simulink model "untitled"  (R2019a)
settings: Solver=VariableStepAuto  StartTime=0.0  StopTime=1  RelTol=1e-3
values from neighbouring files (symbols this model uses):
  Ts_Control = 5.0000e-05    (= 5e-05)    [Sec_Impedance.m]
  Ts_Power = 5.0000e-05    (= 5e-05)    [Sec_Impedance.m]
undefined symbols (not defined in the file or in its folder): D1, Delta, Ion, Lithium
libraries: powerlib x152, powerlib_meascontrol x65, simulink x14, electricdrivelib x12, simulink_extras x12
(part 2 of 5)

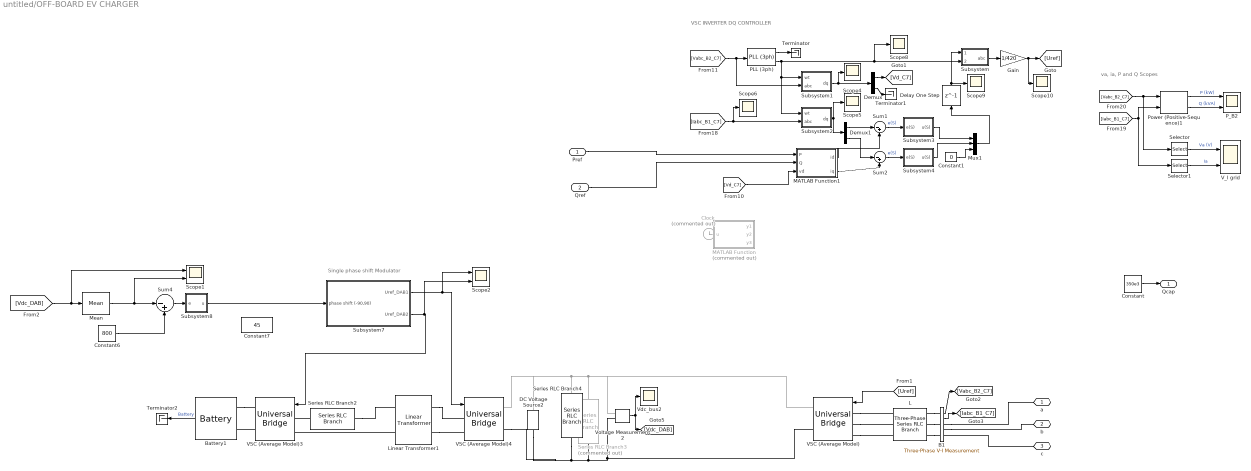
== system untitled/OFF-BOARD EV CHARGER ==
  note: VSC INVERTER DQ CONTROLLER
  note: va, ia, P and Q Scopes
  note: Single phase shift Modulator
  Pref : Inport
  Qref : Inport  Port=2
  B1 : powerlib/Measurements/Three-Phase V-I Measurement  VoltageMeasurement=phase-to-ground  SetLabelV=off  LabelV=Vabc_B1  Vpu=off  VpuLL=off  CurrentMeasurement=yes  SetLabelI=off  LabelI=Iabc_B1_C7  Ipu=off  Pbase=100e6  Vbase=500e3  OutputType=Magnitude  PhasorSimulation=off  PSBequivalent=0
      settings: SourceProductName=Simscape Electrical
  Battery1 : electricdrivelib/Extra Sources/Battery  BatType=Lithium-Ion  ShowTempParam=off  ThermalPreset=no  ShowAgeParam=off  NomV=380  NomQ=5.4*70  SOC=70  Batt_Tr=20  PresetModel=on  MaxQ=378  MinV=285  FullV=442.3151  Dis_rate=164.3478  R=0.010053  Normal_OP=341.8435  expZone="[410.5466       18.5713]"  current=[6.5 13 32.5]  Units=Time  Tci=20  NomT=20  T2=-30  MaxQ2=4.8  FullV2=7.1  Normal_OP2=5.655  expZone2="[6.58           1]"  Rca=0.6  ti=2000  Dp=0  Neq0=0  Tsim=1e6  Ta1=25  Qeol=5.4*0.9  Reol=0.013333*1.2  Char_age=[2.3478, 3]  Dis_age=[2.3478, 10]  N1=1500  N2=10500  N3=1000  N4=1400  Ta2=45  N5=950
      settings: SourceProductName=Simscape Electrical
  Clock : Clock  Commented=on
  Constant : Constant  Value=350e3
  Constant1 : Constant  Value=0
  Constant6 : Constant  Value=800
  Constant7 : Constant  Value=45
  DC Voltage Source2 : powerlib/Electrical Sources/DC Voltage Source  Amplitude=Vdc  Measurements=None
      settings: SourceProductName=Simscape Electrical
  Delay One Step : Delay  DelayLength=1
  Demux : Demux  Outputs=2
  Demux1 : Demux  Outputs=2
  Gain : Gain  Gain=1/420
  L : powerlib/Elements/Three-Phase Series RLC Branch  LConnTagsString=A|B|C  RConnTagsString=A|B|C  BranchType=RL  Resistance=500e-6*377/50/2  Inductance=1200e-6/2  Capacitance=inf  Measurements=None
      settings: SourceProductName=Simscape Electrical
  Linear Transformer1 : powerlib/Elements/Linear Transformer  UNITS=SI  NominalPower=[ 250e3 10000 ]  winding1=[400 0.0032 0.4883e-06]  winding2=[800 0.0032 0.4883e-06]  ThreeWindings=off  winding3=[3.15e+05 19845 2105.6]  RmLm=[800 2.1221]  Measurements=None  DataType=on
      settings: SourceProductName=Simscape Electrical
  MATLAB Function : MATLAB Function  Commented=on  TreatAsAtomicUnit=on
  MATLAB Function1 : MATLAB Function  TreatAsAtomicUnit=on
  Mean : powerlib_meascontrol/Measurements/Mean  Freq=300  Vinit=800  Ts=0
      settings: SourceProductName=Simscape Electrical
  Mux1 : Mux  Inputs=3
  PLL (3ph) : powerlib_meascontrol/PLL/PLL (3ph)  Fmin=58  Par_Init="[-0.57  60]"  ParK=[180, 3200, 1]  TcD=1e-4  MaxRateChangeFreq=12  FilterCutOffFreq=25  Ts=Ts  AGC=on
      settings: SourceProductName=Simscape Electrical
  P_B2 : Scope  NumInputPorts=2
  Power (Positive-Sequence)1 : powerlib_meascontrol/Measurements/Power (Positive-Sequence)  Freq=60  Vinit=[0, 0]  Iinit=[0, 0]  Ts=Ts
      settings: SourceProductName=Simscape Electrical  SourceProductBaseCode=PS
  Scope1 : Scope  NumInputPorts=2
  Scope{4..6,8..10} (6 alike) : Scope
  Scope2 : Scope  NumInputPorts=2
  Selector : Selector  InputPortWidth=3  IndexOptions=Index vector (dialog)  Indices=[1]  OutputSizes=1
  Selector1 : Selector  InputPortWidth=3  IndexOptions=Index vector (dialog)  Indices=[1]  OutputSizes=1
  Series RLC Branch2 : powerlib/Elements/Series RLC Branch  LConnTagsString=__new0  RConnTagsString=__new0  BranchType=L  Resistance=1  Inductance=15e-6  SetiL0=off  InitialCurrent=0  Capacitance=1e-6  Setx0=off  InitialVoltage=0  Measurements=None
      settings: SourceProductName=Simscape Electrical
  Series RLC Branch3 : powerlib/Elements/Series RLC Branch  Commented=on  LConnTagsString=__new0  RConnTagsString=__new0  BranchType=R  Resistance=10  Inductance=1e-3  SetiL0=off  InitialCurrent=0  Capacitance=C  Setx0=off  InitialVoltage=400  Measurements=None
      settings: SourceProductName=Simscape Electrical
  Series RLC Branch4 : powerlib/Elements/Series RLC Branch  LConnTagsString=__new0  RConnTagsString=__new0  BranchType=RC  Resistance=0.1  Inductance=1e-3  SetiL0=off  InitialCurrent=0  Capacitance=C  Setx0=off  InitialVoltage=400  Measurements=None
      settings: SourceProductName=Simscape Electrical
  Subsystem : Subsystem
  Subsystem1 : Subsystem
  Subsystem2 : Subsystem
  Subsystem3 : Subsystem
  Subsystem4 : Subsystem
  Subsystem7 : Subsystem
  Subsystem8 : Subsystem
  Sum1 : Sum  Inputs=|-+
  Sum2 : Sum  Inputs=|-+
  Sum4 : Sum  Inputs=|-+
  Terminator : Terminator
  Terminator1 : Terminator
  Terminator2 : Terminator
  VSC (Average Model) : powerlib/Power Electronics/Universal Bridge  Arms=3  SnubberResistance=1e5  SnubberCapacitance=inf  Device=Average-model based VSC  Ron=1e-3  Lon=0  ForwardVoltages="[  0  0  ]"  ForwardVoltage=0  GTOparameters=[ 10e-6 , 20e-6 ]  IGBTparameters=[ 1e-6 , 2e-6 ]  Measurements=None  Measurements_2=None  converterType=Rectifier
      settings: SourceProductName=Simscape Electrical
  VSC (Average Model)3 : powerlib/Power Electronics/Universal Bridge  Arms=2  SnubberResistance=1e5  SnubberCapacitance=inf  Device=Average-model based VSC  Ron=1e-3  Lon=0  ForwardVoltages="[  0  0  ]"  ForwardVoltage=0  GTOparameters=[ 10e-6 , 20e-6 ]  IGBTparameters=[ 1e-6 , 2e-6 ]  Measurements=None  Measurements_2=None  converterType=Rectifier
      settings: SourceProductName=Simscape Electrical
  VSC (Average Model)4 : powerlib/Power Electronics/Universal Bridge  Arms=2  SnubberResistance=1e5  SnubberCapacitance=inf  Device=Average-model based VSC  Ron=1e-3  Lon=0  ForwardVoltages="[  0  0  ]"  ForwardVoltage=0  GTOparameters=[ 10e-6 , 20e-6 ]  IGBTparameters=[ 1e-6 , 2e-6 ]  Measurements=None  Measurements_2=None  converterType=Rectifier
      settings: SourceProductName=Simscape Electrical
  V_I grid : Scope  NumInputPorts=2
  Vdc_bus2 : Scope
  Voltage Measurement2 : powerlib/Measurements/Voltage Measurement  PhasorSimulation=off  OutputType=Complex  PSBequivalent=0
      settings: SourceProductName=Simscape Electrical
  a : PMIOPort  Side=Right
  b : PMIOPort  Port=2  Side=Right
  c : PMIOPort  Port=3  Side=Right
  Qcap : Outport
  wires:
  Sum2/1 -> Subsystem4/1(e(S))  "e(S)"
  PLL (3ph)/2 -> Subsystem2/1(wt), Subsystem1/1(wt), Scope8/1, Subsystem/2(wt1)
  Mux1/1 -> Delay One Step/1
  Selector/1 -> V_I grid/1  "Va (V)"
  Delay One Step/1 -> Scope9/1, Subsystem/1(dq0)
  MATLAB Function1/1(id) -> Sum1/2
  Sum1/1 -> Subsystem3/1(e(S))  "e(S)"
  Subsystem4/1(u(S)) -> Mux1/2
  Power (Positive-Sequence)1/2 -> P_B2/2  "Q (kVA)"
  Demux/1 -> [Vd_C7]
  Pref/1 -> MATLAB Function1/1(P)
  [Iabc_B1_C7] -> Scope6/1, Subsystem2/2(abc)
  Subsystem/1(abc) -> Gain/1
  [Vabc_B2_C7] -> Selector/1, Power (Positive-Sequence)1/1
  Subsystem3/1(u(S)) -> Mux1/1
  Gain/1 -> Scope10/1, [Uref]
  Qref/1 -> MATLAB Function1/2(Q)
  [Vabc_B2_C7] -> Subsystem1/2(abc), PLL (3ph)/1
  Selector1/1 -> V_I grid/2  "Ia"
  Demux1/1 -> Sum1/1
  [Uref] -> VSC (Average Model)/1
  Demux/2 -> Terminator1/1
  [Iabc_B1_C7] -> Power (Positive-Sequence)1/2, Selector1/1
  Constant1/1 -> Mux1/3
  Subsystem1/1(dq) -> Demux/1, Scope4/1
  Demux1/2 -> Sum2/1
  Power (Positive-Sequence)1/1 -> P_B2/1  "P (kW)"
  MATLAB Function1/2(iq) -> Sum2/2
  [Vd_C7] -> MATLAB Function1/3(vd)
  PLL (3ph)/1 -> Terminator/1
  Subsystem2/1(dq) -> Demux1/1, Scope5/1
  B1/1 -> [Vabc_B2_C7]
  B1/2 -> [Iabc_B1_C7]
  Clock/1 -> MATLAB Function/1(u)
  Mean/1 -> Scope1/2, Sum4/1
  Constant6/1 -> Sum4/2
  [Vdc_DAB] -> Scope1/1, Mean/1
  Subsystem7/1(Uref_DAB1) -> Scope2/1, VSC (Average Model)4/1
  Subsystem7/2(Uref_DAB2) -> Scope2/2, VSC (Average Model)3/1
  Voltage Measurement2/1 -> Vdc_bus2/1, [Vdc_DAB]
  Sum4/1 -> Subsystem8/1(e)
  Subsystem8/1(u) -> Subsystem7/1(phase shift (-90,90))
  Battery1/1 -> Terminator2/1  "Battery"
  Constant/1 -> Qcap/1
  connections:
  VSC (Average Model)/LConn3 -- L/LConn3
  L/RConn1 -- B1/LConn1
  VSC (Average Model)/LConn1 -- L/LConn1
  L/RConn2 -- B1/LConn2
  VSC (Average Model)/LConn2 -- L/LConn2
  L/RConn3 -- B1/LConn3
  c/RConn1 -- B1/RConn3
  B1/RConn1 -- a/RConn1
  B1/RConn2 -- b/RConn1
  Series RLC Branch3/LConn1 -- VSC (Average Model)/RConn1 -- Voltage Measurement2/LConn1 -- Series RLC Branch4/LConn1 -- DC Voltage Source2/RConn1 -- VSC (Average Model)4/RConn1
  Voltage Measurement2/LConn2 -- VSC (Average Model)/RConn2 -- Series RLC Branch4/RConn1 -- VSC (Average Model)4/RConn2 -- DC Voltage Source2/LConn1 -- Series RLC Branch3/RConn1
  Linear Transformer1/RConn1 -- VSC (Average Model)4/LConn1
  Battery1/LConn1 -- VSC (Average Model)3/RConn1
  Series RLC Branch2/LConn1 -- VSC (Average Model)3/LConn1
  VSC (Average Model)3/RConn2 -- Battery1/LConn2
  Linear Transformer1/RConn2 -- VSC (Average Model)4/LConn2
  Series RLC Branch2/RConn1 -- Linear Transformer1/LConn1
  Linear Transformer1/LConn2 -- VSC (Average Model)3/LConn2

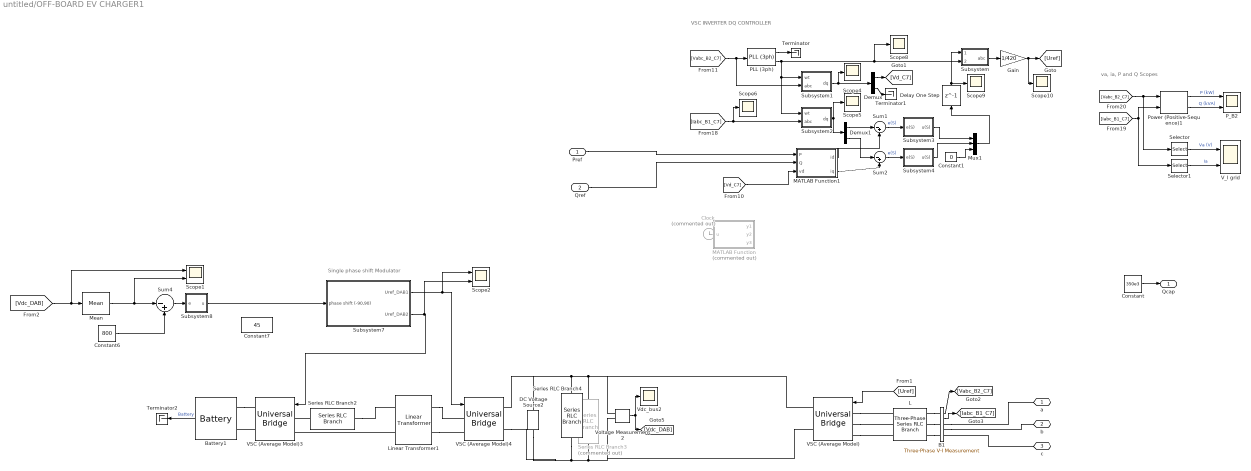
== system untitled/OFF-BOARD EV CHARGER1 ==
  note: VSC INVERTER DQ CONTROLLER
  note: va, ia, P and Q Scopes
  note: Single phase shift Modulator
  Pref : Inport
  Qref : Inport  Port=2
  B1 : powerlib/Measurements/Three-Phase V-I Measurement  VoltageMeasurement=phase-to-ground  SetLabelV=off  LabelV=Vabc_B1  Vpu=off  VpuLL=off  CurrentMeasurement=yes  SetLabelI=off  LabelI=Iabc_B1_C7  Ipu=off  Pbase=100e6  Vbase=500e3  OutputType=Magnitude  PhasorSimulation=off  PSBequivalent=0
      settings: SourceProductName=Simscape Electrical
  Battery1 : electricdrivelib/Extra Sources/Battery  BatType=Lithium-Ion  ShowTempParam=off  ThermalPreset=no  ShowAgeParam=off  NomV=380  NomQ=5.4*70  SOC=70  Batt_Tr=20  PresetModel=on  MaxQ=378  MinV=285  FullV=442.3151  Dis_rate=164.3478  R=0.010053  Normal_OP=341.8435  expZone="[410.5466       18.5713]"  current=[6.5 13 32.5]  Units=Time  Tci=20  NomT=20  T2=-30  MaxQ2=4.8  FullV2=7.1  Normal_OP2=5.655  expZone2="[6.58           1]"  Rca=0.6  ti=2000  Dp=0  Neq0=0  Tsim=1e6  Ta1=25  Qeol=5.4*0.9  Reol=0.013333*1.2  Char_age=[2.3478, 3]  Dis_age=[2.3478, 10]  N1=1500  N2=10500  N3=1000  N4=1400  Ta2=45  N5=950
      settings: SourceProductName=Simscape Electrical
  Clock : Clock  Commented=on
  Constant : Constant  Value=350e3
  Constant1 : Constant  Value=0
  Constant6 : Constant  Value=800
  Constant7 : Constant  Value=45
  DC Voltage Source2 : powerlib/Electrical Sources/DC Voltage Source  Amplitude=Vdc  Measurements=None
      settings: SourceProductName=Simscape Electrical
  Delay One Step : Delay  DelayLength=1
  Demux : Demux  Outputs=2
  Demux1 : Demux  Outputs=2
  Gain : Gain  Gain=1/420
  L : powerlib/Elements/Three-Phase Series RLC Branch  LConnTagsString=A|B|C  RConnTagsString=A|B|C  BranchType=RL  Resistance=500e-6*377/50/2  Inductance=1200e-6/2  Capacitance=inf  Measurements=None
      settings: SourceProductName=Simscape Electrical
  Linear Transformer1 : powerlib/Elements/Linear Transformer  UNITS=SI  NominalPower=[ 250e3 10000 ]  winding1=[400 0.0032 0.4883e-06]  winding2=[800 0.0032 0.4883e-06]  ThreeWindings=off  winding3=[3.15e+05 19845 2105.6]  RmLm=[800 2.1221]  Measurements=None  DataType=on
      settings: SourceProductName=Simscape Electrical
  MATLAB Function : MATLAB Function  Commented=on  TreatAsAtomicUnit=on
  MATLAB Function1 : MATLAB Function  TreatAsAtomicUnit=on
  Mean : powerlib_meascontrol/Measurements/Mean  Freq=300  Vinit=800  Ts=0
      settings: SourceProductName=Simscape Electrical
  Mux1 : Mux  Inputs=3
  PLL (3ph) : powerlib_meascontrol/PLL/PLL (3ph)  Fmin=58  Par_Init="[-0.57  60]"  ParK=[180, 3200, 1]  TcD=1e-4  MaxRateChangeFreq=12  FilterCutOffFreq=25  Ts=Ts  AGC=on
      settings: SourceProductName=Simscape Electrical
  P_B2 : Scope  NumInputPorts=2
  Power (Positive-Sequence)1 : powerlib_meascontrol/Measurements/Power (Positive-Sequence)  Freq=60  Vinit=[0, 0]  Iinit=[0, 0]  Ts=Ts
      settings: SourceProductName=Simscape Electrical  SourceProductBaseCode=PS
  Scope1 : Scope  NumInputPorts=2
  Scope{4..6,8..10} (6 alike) : Scope
  Scope2 : Scope  NumInputPorts=2
  Selector : Selector  InputPortWidth=3  IndexOptions=Index vector (dialog)  Indices=[1]  OutputSizes=1
  Selector1 : Selector  InputPortWidth=3  IndexOptions=Index vector (dialog)  Indices=[1]  OutputSizes=1
  Series RLC Branch2 : powerlib/Elements/Series RLC Branch  LConnTagsString=__new0  RConnTagsString=__new0  BranchType=L  Resistance=1  Inductance=15e-6  SetiL0=off  InitialCurrent=0  Capacitance=1e-6  Setx0=off  InitialVoltage=0  Measurements=None
      settings: SourceProductName=Simscape Electrical
  Series RLC Branch3 : powerlib/Elements/Series RLC Branch  Commented=on  LConnTagsString=__new0  RConnTagsString=__new0  BranchType=R  Resistance=10  Inductance=1e-3  SetiL0=off  InitialCurrent=0  Capacitance=C  Setx0=off  InitialVoltage=400  Measurements=None
      settings: SourceProductName=Simscape Electrical
  Series RLC Branch4 : powerlib/Elements/Series RLC Branch  LConnTagsString=__new0  RConnTagsString=__new0  BranchType=RC  Resistance=0.1  Inductance=1e-3  SetiL0=off  InitialCurrent=0  Capacitance=C  Setx0=off  InitialVoltage=400  Measurements=None
      settings: SourceProductName=Simscape Electrical
  Subsystem : Subsystem
  Subsystem1 : Subsystem
  Subsystem2 : Subsystem
  Subsystem3 : Subsystem
  Subsystem4 : Subsystem
  Subsystem7 : Subsystem
  Subsystem8 : Subsystem
  Sum1 : Sum  Inputs=|-+
  Sum2 : Sum  Inputs=|-+
  Sum4 : Sum  Inputs=|-+
  Terminator : Terminator
  Terminator1 : Terminator
  Terminator2 : Terminator
  VSC (Average Model) : powerlib/Power Electronics/Universal Bridge  Arms=3  SnubberResistance=1e5  SnubberCapacitance=inf  Device=Average-model based VSC  Ron=1e-3  Lon=0  ForwardVoltages="[  0  0  ]"  ForwardVoltage=0  GTOparameters=[ 10e-6 , 20e-6 ]  IGBTparameters=[ 1e-6 , 2e-6 ]  Measurements=None  Measurements_2=None  converterType=Rectifier
      settings: SourceProductName=Simscape Electrical
  VSC (Average Model)3 : powerlib/Power Electronics/Universal Bridge  Arms=2  SnubberResistance=1e5  SnubberCapacitance=inf  Device=Average-model based VSC  Ron=1e-3  Lon=0  ForwardVoltages="[  0  0  ]"  ForwardVoltage=0  GTOparameters=[ 10e-6 , 20e-6 ]  IGBTparameters=[ 1e-6 , 2e-6 ]  Measurements=None  Measurements_2=None  converterType=Rectifier
      settings: SourceProductName=Simscape Electrical
  VSC (Average Model)4 : powerlib/Power Electronics/Universal Bridge  Arms=2  SnubberResistance=1e5  SnubberCapacitance=inf  Device=Average-model based VSC  Ron=1e-3  Lon=0  ForwardVoltages="[  0  0  ]"  ForwardVoltage=0  GTOparameters=[ 10e-6 , 20e-6 ]  IGBTparameters=[ 1e-6 , 2e-6 ]  Measurements=None  Measurements_2=None  converterType=Rectifier
      settings: SourceProductName=Simscape Electrical
  V_I grid : Scope  NumInputPorts=2
  Vdc_bus2 : Scope
  Voltage Measurement2 : powerlib/Measurements/Voltage Measurement  PhasorSimulation=off  OutputType=Complex  PSBequivalent=0
      settings: SourceProductName=Simscape Electrical
  a : PMIOPort  Side=Right
  b : PMIOPort  Port=2  Side=Right
  c : PMIOPort  Port=3  Side=Right
  Qcap : Outport
  wires:
  Sum2/1 -> Subsystem4/1(e(S))  "e(S)"
  PLL (3ph)/2 -> Subsystem2/1(wt), Subsystem1/1(wt), Scope8/1, Subsystem/2(wt1)
  Mux1/1 -> Delay One Step/1
  Selector/1 -> V_I grid/1  "Va (V)"
  Delay One Step/1 -> Scope9/1, Subsystem/1(dq0)
  MATLAB Function1/1(id) -> Sum1/2
  Sum1/1 -> Subsystem3/1(e(S))  "e(S)"
  Subsystem4/1(u(S)) -> Mux1/2
  Power (Positive-Sequence)1/2 -> P_B2/2  "Q (kVA)"
  Demux/1 -> [Vd_C7]
  Pref/1 -> MATLAB Function1/1(P)
  [Iabc_B1_C7] -> Scope6/1, Subsystem2/2(abc)
  Subsystem/1(abc) -> Gain/1
  [Vabc_B2_C7] -> Selector/1, Power (Positive-Sequence)1/1
  Subsystem3/1(u(S)) -> Mux1/1
  Gain/1 -> Scope10/1, [Uref]
  Qref/1 -> MATLAB Function1/2(Q)
  [Vabc_B2_C7] -> Subsystem1/2(abc), PLL (3ph)/1
  Selector1/1 -> V_I grid/2  "Ia"
  Demux1/1 -> Sum1/1
  [Uref] -> VSC (Average Model)/1
  Demux/2 -> Terminator1/1
  [Iabc_B1_C7] -> Power (Positive-Sequence)1/2, Selector1/1
  Constant1/1 -> Mux1/3
  Subsystem1/1(dq) -> Demux/1, Scope4/1
  Demux1/2 -> Sum2/1
  Power (Positive-Sequence)1/1 -> P_B2/1  "P (kW)"
  MATLAB Function1/2(iq) -> Sum2/2
  [Vd_C7] -> MATLAB Function1/3(vd)
  PLL (3ph)/1 -> Terminator/1
  Subsystem2/1(dq) -> Demux1/1, Scope5/1
  B1/1 -> [Vabc_B2_C7]
  B1/2 -> [Iabc_B1_C7]
  Clock/1 -> MATLAB Function/1(u)
  Mean/1 -> Scope1/2, Sum4/1
  Constant6/1 -> Sum4/2
  [Vdc_DAB] -> Scope1/1, Mean/1
  Subsystem7/1(Uref_DAB1) -> Scope2/1, VSC (Average Model)4/1
  Subsystem7/2(Uref_DAB2) -> Scope2/2, VSC (Average Model)3/1
  Voltage Measurement2/1 -> Vdc_bus2/1, [Vdc_DAB]
  Sum4/1 -> Subsystem8/1(e)
  Subsystem8/1(u) -> Subsystem7/1(phase shift (-90,90))
  Battery1/1 -> Terminator2/1  "Battery"
  Constant/1 -> Qcap/1
  connections:
  VSC (Average Model)/LConn3 -- L/LConn3
  L/RConn1 -- B1/LConn1
  VSC (Average Model)/LConn1 -- L/LConn1
  L/RConn2 -- B1/LConn2
  VSC (Average Model)/LConn2 -- L/LConn2
  L/RConn3 -- B1/LConn3
  c/RConn1 -- B1/RConn3
  B1/RConn1 -- a/RConn1
  B1/RConn2 -- b/RConn1
  Series RLC Branch4/LConn1 -- DC Voltage Source2/RConn1 -- VSC (Average Model)4/RConn1 -- Series RLC Branch3/LConn1 -- VSC (Average Model)/RConn1 -- Voltage Measurement2/LConn1
  Series RLC Branch4/RConn1 -- VSC (Average Model)4/RConn2 -- DC Voltage Source2/LConn1 -- Series RLC Branch3/RConn1 -- Voltage Measurement2/LConn2 -- VSC (Average Model)/RConn2
  Linear Transformer1/RConn1 -- VSC (Average Model)4/LConn1
  Battery1/LConn1 -- VSC (Average Model)3/RConn1
  Series RLC Branch2/LConn1 -- VSC (Average Model)3/LConn1
  VSC (Average Model)3/RConn2 -- Battery1/LConn2
  Linear Transformer1/RConn2 -- VSC (Average Model)4/LConn2
  Series RLC Branch2/RConn1 -- Linear Transformer1/LConn1
  Linear Transformer1/LConn2 -- VSC (Average Model)3/LConn2

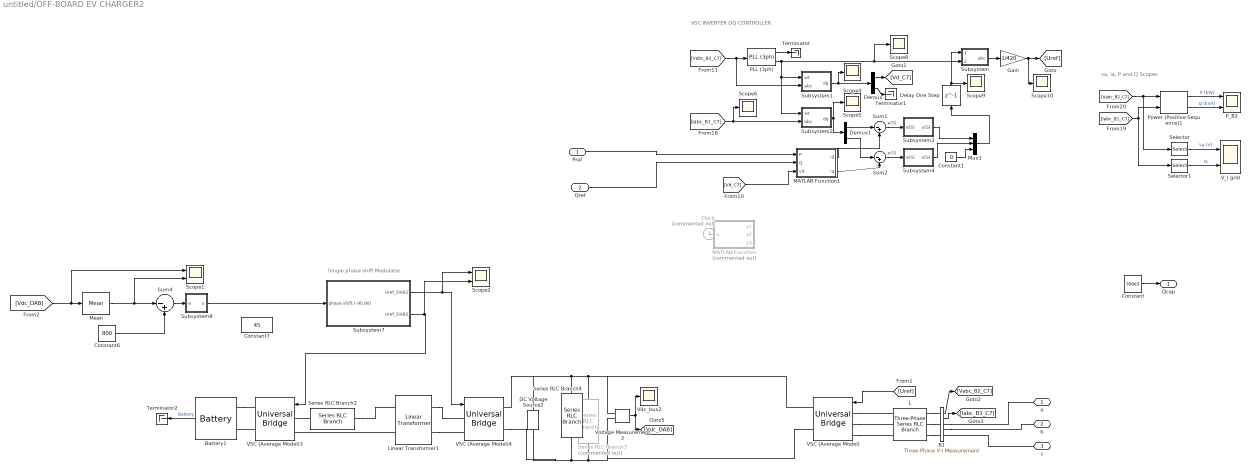
== system untitled/OFF-BOARD EV CHARGER2 ==
  note: VSC INVERTER DQ CONTROLLER
  note: va, ia, P and Q Scopes
  note: Single phase shift Modulator
  Pref : Inport
  Qref : Inport  Port=2
  B1 : powerlib/Measurements/Three-Phase V-I Measurement  VoltageMeasurement=phase-to-ground  SetLabelV=off  LabelV=Vabc_B1  Vpu=off  VpuLL=off  CurrentMeasurement=yes  SetLabelI=off  LabelI=Iabc_B1_C7  Ipu=off  Pbase=100e6  Vbase=500e3  OutputType=Magnitude  PhasorSimulation=off  PSBequivalent=0
      settings: SourceProductName=Simscape Electrical
  Battery1 : electricdrivelib/Extra Sources/Battery  BatType=Lithium-Ion  ShowTempParam=off  ThermalPreset=no  ShowAgeParam=off  NomV=380  NomQ=5.4*70  SOC=70  Batt_Tr=20  PresetModel=on  MaxQ=378  MinV=285  FullV=442.3151  Dis_rate=164.3478  R=0.010053  Normal_OP=341.8435  expZone="[410.5466       18.5713]"  current=[6.5 13 32.5]  Units=Time  Tci=20  NomT=20  T2=-30  MaxQ2=4.8  FullV2=7.1  Normal_OP2=5.655  expZone2="[6.58           1]"  Rca=0.6  ti=2000  Dp=0  Neq0=0  Tsim=1e6  Ta1=25  Qeol=5.4*0.9  Reol=0.013333*1.2  Char_age=[2.3478, 3]  Dis_age=[2.3478, 10]  N1=1500  N2=10500  N3=1000  N4=1400  Ta2=45  N5=950
      settings: SourceProductName=Simscape Electrical
  Clock : Clock  Commented=on
  Constant : Constant  Value=350e3
  Constant1 : Constant  Value=0
  Constant6 : Constant  Value=800
  Constant7 : Constant  Value=45
  DC Voltage Source2 : powerlib/Electrical Sources/DC Voltage Source  Amplitude=Vdc  Measurements=None
      settings: SourceProductName=Simscape Electrical
  Delay One Step : Delay  DelayLength=1
  Demux : Demux  Outputs=2
  Demux1 : Demux  Outputs=2
  Gain : Gain  Gain=1/420
  L : powerlib/Elements/Three-Phase Series RLC Branch  LConnTagsString=A|B|C  RConnTagsString=A|B|C  BranchType=RL  Resistance=500e-6*377/50/2  Inductance=1200e-6/2  Capacitance=inf  Measurements=None
      settings: SourceProductName=Simscape Electrical
  Linear Transformer1 : powerlib/Elements/Linear Transformer  UNITS=SI  NominalPower=[ 250e3 10000 ]  winding1=[400 0.0032 0.4883e-06]  winding2=[800 0.0032 0.4883e-06]  ThreeWindings=off  winding3=[3.15e+05 19845 2105.6]  RmLm=[800 2.1221]  Measurements=None  DataType=on
      settings: SourceProductName=Simscape Electrical
  MATLAB Function : MATLAB Function  Commented=on  TreatAsAtomicUnit=on
  MATLAB Function1 : MATLAB Function  TreatAsAtomicUnit=on
  Mean : powerlib_meascontrol/Measurements/Mean  Freq=300  Vinit=800  Ts=0
      settings: SourceProductName=Simscape Electrical
  Mux1 : Mux  Inputs=3
  PLL (3ph) : powerlib_meascontrol/PLL/PLL (3ph)  Fmin=58  Par_Init="[-0.57  60]"  ParK=[180, 3200, 1]  TcD=1e-4  MaxRateChangeFreq=12  FilterCutOffFreq=25  Ts=Ts  AGC=on
      settings: SourceProductName=Simscape Electrical
  P_B2 : Scope  NumInputPorts=2
  Power (Positive-Sequence)1 : powerlib_meascontrol/Measurements/Power (Positive-Sequence)  Freq=60  Vinit=[0, 0]  Iinit=[0, 0]  Ts=Ts
      settings: SourceProductName=Simscape Electrical  SourceProductBaseCode=PS
  Scope1 : Scope  NumInputPorts=2
  Scope{4..6,8..10} (6 alike) : Scope
  Scope2 : Scope  NumInputPorts=2
  Selector : Selector  InputPortWidth=3  IndexOptions=Index vector (dialog)  Indices=[1]  OutputSizes=1
  Selector1 : Selector  InputPortWidth=3  IndexOptions=Index vector (dialog)  Indices=[1]  OutputSizes=1
  Series RLC Branch2 : powerlib/Elements/Series RLC Branch  LConnTagsString=__new0  RConnTagsString=__new0  BranchType=L  Resistance=1  Inductance=15e-6  SetiL0=off  InitialCurrent=0  Capacitance=1e-6  Setx0=off  InitialVoltage=0  Measurements=None
      settings: SourceProductName=Simscape Electrical
  Series RLC Branch3 : powerlib/Elements/Series RLC Branch  Commented=on  LConnTagsString=__new0  RConnTagsString=__new0  BranchType=R  Resistance=10  Inductance=1e-3  SetiL0=off  InitialCurrent=0  Capacitance=C  Setx0=off  InitialVoltage=400  Measurements=None
      settings: SourceProductName=Simscape Electrical
  Series RLC Branch4 : powerlib/Elements/Series RLC Branch  LConnTagsString=__new0  RConnTagsString=__new0  BranchType=RC  Resistance=0.1  Inductance=1e-3  SetiL0=off  InitialCurrent=0  Capacitance=C  Setx0=off  InitialVoltage=400  Measurements=None
      settings: SourceProductName=Simscape Electrical
  Subsystem : Subsystem
  Subsystem1 : Subsystem
  Subsystem2 : Subsystem
  Subsystem3 : Subsystem
  Subsystem4 : Subsystem
  Subsystem7 : Subsystem
  Subsystem8 : Subsystem
  Sum1 : Sum  Inputs=|-+
  Sum2 : Sum  Inputs=|-+
  Sum4 : Sum  Inputs=|-+
  Terminator : Terminator
  Terminator1 : Terminator
  Terminator2 : Terminator
  VSC (Average Model) : powerlib/Power Electronics/Universal Bridge  Arms=3  SnubberResistance=1e5  SnubberCapacitance=inf  Device=Average-model based VSC  Ron=1e-3  Lon=0  ForwardVoltages="[  0  0  ]"  ForwardVoltage=0  GTOparameters=[ 10e-6 , 20e-6 ]  IGBTparameters=[ 1e-6 , 2e-6 ]  Measurements=None  Measurements_2=None  converterType=Rectifier
      settings: SourceProductName=Simscape Electrical
  VSC (Average Model)3 : powerlib/Power Electronics/Universal Bridge  Arms=2  SnubberResistance=1e5  SnubberCapacitance=inf  Device=Average-model based VSC  Ron=1e-3  Lon=0  ForwardVoltages="[  0  0  ]"  ForwardVoltage=0  GTOparameters=[ 10e-6 , 20e-6 ]  IGBTparameters=[ 1e-6 , 2e-6 ]  Measurements=None  Measurements_2=None  converterType=Rectifier
      settings: SourceProductName=Simscape Electrical
  VSC (Average Model)4 : powerlib/Power Electronics/Universal Bridge  Arms=2  SnubberResistance=1e5  SnubberCapacitance=inf  Device=Average-model based VSC  Ron=1e-3  Lon=0  ForwardVoltages="[  0  0  ]"  ForwardVoltage=0  GTOparameters=[ 10e-6 , 20e-6 ]  IGBTparameters=[ 1e-6 , 2e-6 ]  Measurements=None  Measurements_2=None  converterType=Rectifier
      settings: SourceProductName=Simscape Electrical
  V_I grid : Scope  NumInputPorts=2
  Vdc_bus2 : Scope
  Voltage Measurement2 : powerlib/Measurements/Voltage Measurement  PhasorSimulation=off  OutputType=Complex  PSBequivalent=0
      settings: SourceProductName=Simscape Electrical
  a : PMIOPort  Side=Right
  b : PMIOPort  Port=2  Side=Right
  c : PMIOPort  Port=3  Side=Right
  Qcap : Outport
  wires:
  Sum2/1 -> Subsystem4/1(e(S))  "e(S)"
  PLL (3ph)/2 -> Subsystem2/1(wt), Subsystem1/1(wt), Scope8/1, Subsystem/2(wt1)
  Mux1/1 -> Delay One Step/1
  Selector/1 -> V_I grid/1  "Va (V)"
  Delay One Step/1 -> Scope9/1, Subsystem/1(dq0)
  MATLAB Function1/1(id) -> Sum1/2
  Sum1/1 -> Subsystem3/1(e(S))  "e(S)"
  Subsystem4/1(u(S)) -> Mux1/2
  Power (Positive-Sequence)1/2 -> P_B2/2  "Q (kVA)"
  Demux/1 -> [Vd_C7]
  Pref/1 -> MATLAB Function1/1(P)
  [Iabc_B1_C7] -> Scope6/1, Subsystem2/2(abc)
  Subsystem/1(abc) -> Gain/1
  [Vabc_B2_C7] -> Selector/1, Power (Positive-Sequence)1/1
  Subsystem3/1(u(S)) -> Mux1/1
  Gain/1 -> Scope10/1, [Uref]
  Qref/1 -> MATLAB Function1/2(Q)
  [Vabc_B2_C7] -> Subsystem1/2(abc), PLL (3ph)/1
  Selector1/1 -> V_I grid/2  "Ia"
  Demux1/1 -> Sum1/1
  [Uref] -> VSC (Average Model)/1
  Demux/2 -> Terminator1/1
  [Iabc_B1_C7] -> Power (Positive-Sequence)1/2, Selector1/1
  Constant1/1 -> Mux1/3
  Subsystem1/1(dq) -> Demux/1, Scope4/1
  Demux1/2 -> Sum2/1
  Power (Positive-Sequence)1/1 -> P_B2/1  "P (kW)"
  MATLAB Function1/2(iq) -> Sum2/2
  [Vd_C7] -> MATLAB Function1/3(vd)
  PLL (3ph)/1 -> Terminator/1
  Subsystem2/1(dq) -> Demux1/1, Scope5/1
  B1/1 -> [Vabc_B2_C7]
  B1/2 -> [Iabc_B1_C7]
  Clock/1 -> MATLAB Function/1(u)
  Mean/1 -> Scope1/2, Sum4/1
  Constant6/1 -> Sum4/2
  [Vdc_DAB] -> Scope1/1, Mean/1
  Subsystem7/1(Uref_DAB1) -> Scope2/1, VSC (Average Model)4/1
  Subsystem7/2(Uref_DAB2) -> Scope2/2, VSC (Average Model)3/1
  Voltage Measurement2/1 -> Vdc_bus2/1, [Vdc_DAB]
  Sum4/1 -> Subsystem8/1(e)
  Subsystem8/1(u) -> Subsystem7/1(phase shift (-90,90))
  Battery1/1 -> Terminator2/1  "Battery"
  Constant/1 -> Qcap/1
  connections:
  VSC (Average Model)/LConn3 -- L/LConn3
  L/RConn1 -- B1/LConn1
  VSC (Average Model)/LConn1 -- L/LConn1
  L/RConn2 -- B1/LConn2
  VSC (Average Model)/LConn2 -- L/LConn2
  L/RConn3 -- B1/LConn3
  c/RConn1 -- B1/RConn3
  B1/RConn1 -- a/RConn1
  B1/RConn2 -- b/RConn1
  Series RLC Branch4/LConn1 -- DC Voltage Source2/RConn1 -- VSC (Average Model)4/RConn1 -- Series RLC Branch3/LConn1 -- VSC (Average Model)/RConn1 -- Voltage Measurement2/LConn1
  Series RLC Branch4/RConn1 -- VSC (Average Model)4/RConn2 -- DC Voltage Source2/LConn1 -- Series RLC Branch3/RConn1 -- Voltage Measurement2/LConn2 -- VSC (Average Model)/RConn2
  Linear Transformer1/RConn1 -- VSC (Average Model)4/LConn1
  Battery1/LConn1 -- VSC (Average Model)3/RConn1
  Series RLC Branch2/LConn1 -- VSC (Average Model)3/LConn1
  VSC (Average Model)3/RConn2 -- Battery1/LConn2
  Linear Transformer1/RConn2 -- VSC (Average Model)4/LConn2
  Series RLC Branch2/RConn1 -- Linear Transformer1/LConn1
  Linear Transformer1/LConn2 -- VSC (Average Model)3/LConn2

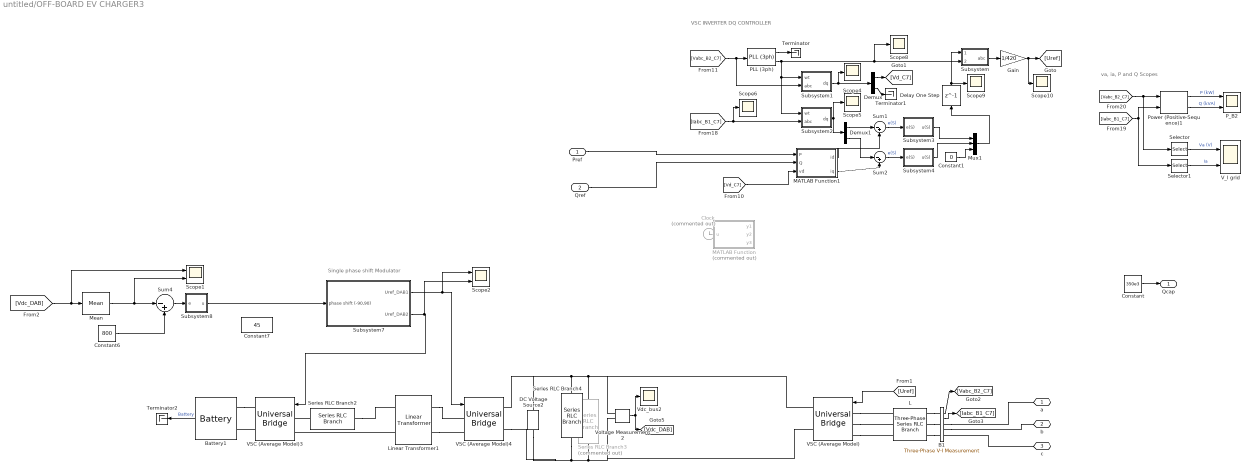
== system untitled/OFF-BOARD EV CHARGER3 ==
  note: VSC INVERTER DQ CONTROLLER
  note: va, ia, P and Q Scopes
  note: Single phase shift Modulator
  Pref : Inport
  Qref : Inport  Port=2
  B1 : powerlib/Measurements/Three-Phase V-I Measurement  VoltageMeasurement=phase-to-ground  SetLabelV=off  LabelV=Vabc_B1  Vpu=off  VpuLL=off  CurrentMeasurement=yes  SetLabelI=off  LabelI=Iabc_B1_C7  Ipu=off  Pbase=100e6  Vbase=500e3  OutputType=Magnitude  PhasorSimulation=off  PSBequivalent=0
      settings: SourceProductName=Simscape Electrical
  Battery1 : electricdrivelib/Extra Sources/Battery  BatType=Lithium-Ion  ShowTempParam=off  ThermalPreset=no  ShowAgeParam=off  NomV=380  NomQ=5.4*70  SOC=70  Batt_Tr=20  PresetModel=on  MaxQ=378  MinV=285  FullV=442.3151  Dis_rate=164.3478  R=0.010053  Normal_OP=341.8435  expZone="[410.5466       18.5713]"  current=[6.5 13 32.5]  Units=Time  Tci=20  NomT=20  T2=-30  MaxQ2=4.8  FullV2=7.1  Normal_OP2=5.655  expZone2="[6.58           1]"  Rca=0.6  ti=2000  Dp=0  Neq0=0  Tsim=1e6  Ta1=25  Qeol=5.4*0.9  Reol=0.013333*1.2  Char_age=[2.3478, 3]  Dis_age=[2.3478, 10]  N1=1500  N2=10500  N3=1000  N4=1400  Ta2=45  N5=950
      settings: SourceProductName=Simscape Electrical
  Clock : Clock  Commented=on
  Constant : Constant  Value=350e3
  Constant1 : Constant  Value=0
  Constant6 : Constant  Value=800
  Constant7 : Constant  Value=45
  DC Voltage Source2 : powerlib/Electrical Sources/DC Voltage Source  Amplitude=Vdc  Measurements=None
      settings: SourceProductName=Simscape Electrical
  Delay One Step : Delay  DelayLength=1
  Demux : Demux  Outputs=2
  Demux1 : Demux  Outputs=2
  Gain : Gain  Gain=1/420
  L : powerlib/Elements/Three-Phase Series RLC Branch  LConnTagsString=A|B|C  RConnTagsString=A|B|C  BranchType=RL  Resistance=500e-6*377/50/2  Inductance=1200e-6/2  Capacitance=inf  Measurements=None
      settings: SourceProductName=Simscape Electrical
  Linear Transformer1 : powerlib/Elements/Linear Transformer  UNITS=SI  NominalPower=[ 250e3 10000 ]  winding1=[400 0.0032 0.4883e-06]  winding2=[800 0.0032 0.4883e-06]  ThreeWindings=off  winding3=[3.15e+05 19845 2105.6]  RmLm=[800 2.1221]  Measurements=None  DataType=on
      settings: SourceProductName=Simscape Electrical
  MATLAB Function : MATLAB Function  Commented=on  TreatAsAtomicUnit=on
  MATLAB Function1 : MATLAB Function  TreatAsAtomicUnit=on
  Mean : powerlib_meascontrol/Measurements/Mean  Freq=300  Vinit=800  Ts=0
      settings: SourceProductName=Simscape Electrical
  Mux1 : Mux  Inputs=3
  PLL (3ph) : powerlib_meascontrol/PLL/PLL (3ph)  Fmin=58  Par_Init="[-0.57  60]"  ParK=[180, 3200, 1]  TcD=1e-4  MaxRateChangeFreq=12  FilterCutOffFreq=25  Ts=Ts  AGC=on
      settings: SourceProductName=Simscape Electrical
  P_B2 : Scope  NumInputPorts=2
  Power (Positive-Sequence)1 : powerlib_meascontrol/Measurements/Power (Positive-Sequence)  Freq=60  Vinit=[0, 0]  Iinit=[0, 0]  Ts=Ts
      settings: SourceProductName=Simscape Electrical  SourceProductBaseCode=PS
  Scope1 : Scope  NumInputPorts=2
  Scope{4..6,8..10} (6 alike) : Scope
  Scope2 : Scope  NumInputPorts=2
  Selector : Selector  InputPortWidth=3  IndexOptions=Index vector (dialog)  Indices=[1]  OutputSizes=1
  Selector1 : Selector  InputPortWidth=3  IndexOptions=Index vector (dialog)  Indices=[1]  OutputSizes=1
  Series RLC Branch2 : powerlib/Elements/Series RLC Branch  LConnTagsString=__new0  RConnTagsString=__new0  BranchType=L  Resistance=1  Inductance=15e-6  SetiL0=off  InitialCurrent=0  Capacitance=1e-6  Setx0=off  InitialVoltage=0  Measurements=None
      settings: SourceProductName=Simscape Electrical
  Series RLC Branch3 : powerlib/Elements/Series RLC Branch  Commented=on  LConnTagsString=__new0  RConnTagsString=__new0  BranchType=R  Resistance=10  Inductance=1e-3  SetiL0=off  InitialCurrent=0  Capacitance=C  Setx0=off  InitialVoltage=400  Measurements=None
      settings: SourceProductName=Simscape Electrical
  Series RLC Branch4 : powerlib/Elements/Series RLC Branch  LConnTagsString=__new0  RConnTagsString=__new0  BranchType=RC  Resistance=0.1  Inductance=1e-3  SetiL0=off  InitialCurrent=0  Capacitance=C  Setx0=off  InitialVoltage=400  Measurements=None
      settings: SourceProductName=Simscape Electrical
  Subsystem : Subsystem
  Subsystem1 : Subsystem
  Subsystem2 : Subsystem
  Subsystem3 : Subsystem
  Subsystem4 : Subsystem
  Subsystem7 : Subsystem
  Subsystem8 : Subsystem
  Sum1 : Sum  Inputs=|-+
  Sum2 : Sum  Inputs=|-+
  Sum4 : Sum  Inputs=|-+
  Terminator : Terminator
  Terminator1 : Terminator
  Terminator2 : Terminator
  VSC (Average Model) : powerlib/Power Electronics/Universal Bridge  Arms=3  SnubberResistance=1e5  SnubberCapacitance=inf  Device=Average-model based VSC  Ron=1e-3  Lon=0  ForwardVoltages="[  0  0  ]"  ForwardVoltage=0  GTOparameters=[ 10e-6 , 20e-6 ]  IGBTparameters=[ 1e-6 , 2e-6 ]  Measurements=None  Measurements_2=None  converterType=Rectifier
      settings: SourceProductName=Simscape Electrical
  VSC (Average Model)3 : powerlib/Power Electronics/Universal Bridge  Arms=2  SnubberResistance=1e5  SnubberCapacitance=inf  Device=Average-model based VSC  Ron=1e-3  Lon=0  ForwardVoltages="[  0  0  ]"  ForwardVoltage=0  GTOparameters=[ 10e-6 , 20e-6 ]  IGBTparameters=[ 1e-6 , 2e-6 ]  Measurements=None  Measurements_2=None  converterType=Rectifier
      settings: SourceProductName=Simscape Electrical
  VSC (Average Model)4 : powerlib/Power Electronics/Universal Bridge  Arms=2  SnubberResistance=1e5  SnubberCapacitance=inf  Device=Average-model based VSC  Ron=1e-3  Lon=0  ForwardVoltages="[  0  0  ]"  ForwardVoltage=0  GTOparameters=[ 10e-6 , 20e-6 ]  IGBTparameters=[ 1e-6 , 2e-6 ]  Measurements=None  Measurements_2=None  converterType=Rectifier
      settings: SourceProductName=Simscape Electrical
  V_I grid : Scope  NumInputPorts=2
  Vdc_bus2 : Scope
  Voltage Measurement2 : powerlib/Measurements/Voltage Measurement  PhasorSimulation=off  OutputType=Complex  PSBequivalent=0
      settings: SourceProductName=Simscape Electrical
  a : PMIOPort  Side=Right
  b : PMIOPort  Port=2  Side=Right
  c : PMIOPort  Port=3  Side=Right
  Qcap : Outport
  wires:
  Sum2/1 -> Subsystem4/1(e(S))  "e(S)"
  PLL (3ph)/2 -> Subsystem2/1(wt), Subsystem1/1(wt), Scope8/1, Subsystem/2(wt1)
  Mux1/1 -> Delay One Step/1
  Selector/1 -> V_I grid/1  "Va (V)"
  Delay One Step/1 -> Scope9/1, Subsystem/1(dq0)
  MATLAB Function1/1(id) -> Sum1/2
  Sum1/1 -> Subsystem3/1(e(S))  "e(S)"
  Subsystem4/1(u(S)) -> Mux1/2
  Power (Positive-Sequence)1/2 -> P_B2/2  "Q (kVA)"
  Demux/1 -> [Vd_C7]
  Pref/1 -> MATLAB Function1/1(P)
  [Iabc_B1_C7] -> Scope6/1, Subsystem2/2(abc)
  Subsystem/1(abc) -> Gain/1
  [Vabc_B2_C7] -> Selector/1, Power (Positive-Sequence)1/1
  Subsystem3/1(u(S)) -> Mux1/1
  Gain/1 -> Scope10/1, [Uref]
  Qref/1 -> MATLAB Function1/2(Q)
  [Vabc_B2_C7] -> Subsystem1/2(abc), PLL (3ph)/1
  Selector1/1 -> V_I grid/2  "Ia"
  Demux1/1 -> Sum1/1
  [Uref] -> VSC (Average Model)/1
  Demux/2 -> Terminator1/1
  [Iabc_B1_C7] -> Power (Positive-Sequence)1/2, Selector1/1
  Constant1/1 -> Mux1/3
  Subsystem1/1(dq) -> Demux/1, Scope4/1
  Demux1/2 -> Sum2/1
  Power (Positive-Sequence)1/1 -> P_B2/1  "P (kW)"
  MATLAB Function1/2(iq) -> Sum2/2
  [Vd_C7] -> MATLAB Function1/3(vd)
  PLL (3ph)/1 -> Terminator/1
  Subsystem2/1(dq) -> Demux1/1, Scope5/1
  B1/1 -> [Vabc_B2_C7]
  B1/2 -> [Iabc_B1_C7]
  Clock/1 -> MATLAB Function/1(u)
  Mean/1 -> Scope1/2, Sum4/1
  Constant6/1 -> Sum4/2
  [Vdc_DAB] -> Scope1/1, Mean/1
  Subsystem7/1(Uref_DAB1) -> Scope2/1, VSC (Average Model)4/1
  Subsystem7/2(Uref_DAB2) -> Scope2/2, VSC (Average Model)3/1
  Voltage Measurement2/1 -> Vdc_bus2/1, [Vdc_DAB]
  Sum4/1 -> Subsystem8/1(e)
  Subsystem8/1(u) -> Subsystem7/1(phase shift (-90,90))
  Battery1/1 -> Terminator2/1  "Battery"
  Constant/1 -> Qcap/1
  connections:
  VSC (Average Model)/LConn3 -- L/LConn3
  L/RConn1 -- B1/LConn1
  VSC (Average Model)/LConn1 -- L/LConn1
  L/RConn2 -- B1/LConn2
  VSC (Average Model)/LConn2 -- L/LConn2
  L/RConn3 -- B1/LConn3
  c/RConn1 -- B1/RConn3
  B1/RConn1 -- a/RConn1
  B1/RConn2 -- b/RConn1
  Series RLC Branch4/LConn1 -- DC Voltage Source2/RConn1 -- VSC (Average Model)4/RConn1 -- Series RLC Branch3/LConn1 -- VSC (Average Model)/RConn1 -- Voltage Measurement2/LConn1
  Series RLC Branch4/RConn1 -- VSC (Average Model)4/RConn2 -- DC Voltage Source2/LConn1 -- Series RLC Branch3/RConn1 -- Voltage Measurement2/LConn2 -- VSC (Average Model)/RConn2
  Linear Transformer1/RConn1 -- VSC (Average Model)4/LConn1
  Battery1/LConn1 -- VSC (Average Model)3/RConn1
  Series RLC Branch2/LConn1 -- VSC (Average Model)3/LConn1
  VSC (Average Model)3/RConn2 -- Battery1/LConn2
  Linear Transformer1/RConn2 -- VSC (Average Model)4/LConn2
  Series RLC Branch2/RConn1 -- Linear Transformer1/LConn1
  Linear Transformer1/LConn2 -- VSC (Average Model)3/LConn2

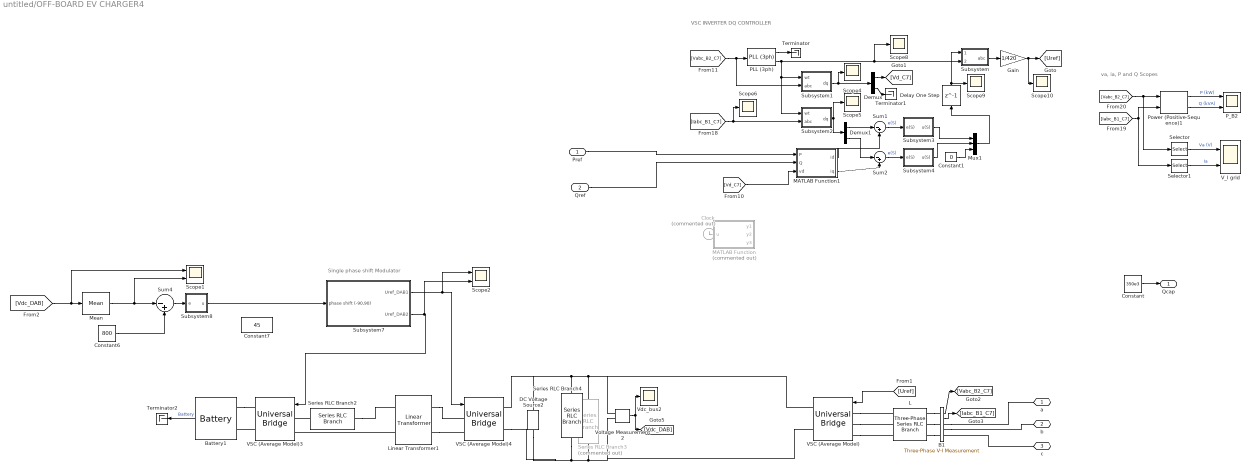
== system untitled/OFF-BOARD EV CHARGER4 ==
  note: VSC INVERTER DQ CONTROLLER
  note: va, ia, P and Q Scopes
  note: Single phase shift Modulator
  Pref : Inport
  Qref : Inport  Port=2
  B1 : powerlib/Measurements/Three-Phase V-I Measurement  VoltageMeasurement=phase-to-ground  SetLabelV=off  LabelV=Vabc_B1  Vpu=off  VpuLL=off  CurrentMeasurement=yes  SetLabelI=off  LabelI=Iabc_B1_C7  Ipu=off  Pbase=100e6  Vbase=500e3  OutputType=Magnitude  PhasorSimulation=off  PSBequivalent=0
      settings: SourceProductName=Simscape Electrical
  Battery1 : electricdrivelib/Extra Sources/Battery  BatType=Lithium-Ion  ShowTempParam=off  ThermalPreset=no  ShowAgeParam=off  NomV=380  NomQ=5.4*70  SOC=70  Batt_Tr=20  PresetModel=on  MaxQ=378  MinV=285  FullV=442.3151  Dis_rate=164.3478  R=0.010053  Normal_OP=341.8435  expZone="[410.5466       18.5713]"  current=[6.5 13 32.5]  Units=Time  Tci=20  NomT=20  T2=-30  MaxQ2=4.8  FullV2=7.1  Normal_OP2=5.655  expZone2="[6.58           1]"  Rca=0.6  ti=2000  Dp=0  Neq0=0  Tsim=1e6  Ta1=25  Qeol=5.4*0.9  Reol=0.013333*1.2  Char_age=[2.3478, 3]  Dis_age=[2.3478, 10]  N1=1500  N2=10500  N3=1000  N4=1400  Ta2=45  N5=950
      settings: SourceProductName=Simscape Electrical
  Clock : Clock  Commented=on
  Constant : Constant  Value=350e3
  Constant1 : Constant  Value=0
  Constant6 : Constant  Value=800
  Constant7 : Constant  Value=45
  DC Voltage Source2 : powerlib/Electrical Sources/DC Voltage Source  Amplitude=Vdc  Measurements=None
      settings: SourceProductName=Simscape Electrical
  Delay One Step : Delay  DelayLength=1
  Demux : Demux  Outputs=2
  Demux1 : Demux  Outputs=2
  Gain : Gain  Gain=1/420
  L : powerlib/Elements/Three-Phase Series RLC Branch  LConnTagsString=A|B|C  RConnTagsString=A|B|C  BranchType=RL  Resistance=500e-6*377/50/2  Inductance=1200e-6/2  Capacitance=inf  Measurements=None
      settings: SourceProductName=Simscape Electrical
  Linear Transformer1 : powerlib/Elements/Linear Transformer  UNITS=SI  NominalPower=[ 250e3 10000 ]  winding1=[400 0.0032 0.4883e-06]  winding2=[800 0.0032 0.4883e-06]  ThreeWindings=off  winding3=[3.15e+05 19845 2105.6]  RmLm=[800 2.1221]  Measurements=None  DataType=on
      settings: SourceProductName=Simscape Electrical
  MATLAB Function : MATLAB Function  Commented=on  TreatAsAtomicUnit=on
  MATLAB Function1 : MATLAB Function  TreatAsAtomicUnit=on
  Mean : powerlib_meascontrol/Measurements/Mean  Freq=300  Vinit=800  Ts=0
      settings: SourceProductName=Simscape Electrical
  Mux1 : Mux  Inputs=3
  PLL (3ph) : powerlib_meascontrol/PLL/PLL (3ph)  Fmin=58  Par_Init="[-0.57  60]"  ParK=[180, 3200, 1]  TcD=1e-4  MaxRateChangeFreq=12  FilterCutOffFreq=25  Ts=Ts  AGC=on
      settings: SourceProductName=Simscape Electrical
  P_B2 : Scope  NumInputPorts=2
  Power (Positive-Sequence)1 : powerlib_meascontrol/Measurements/Power (Positive-Sequence)  Freq=60  Vinit=[0, 0]  Iinit=[0, 0]  Ts=Ts
      settings: SourceProductName=Simscape Electrical  SourceProductBaseCode=PS
  Scope1 : Scope  NumInputPorts=2
  Scope{4..6,8..10} (6 alike) : Scope
  Scope2 : Scope  NumInputPorts=2
  Selector : Selector  InputPortWidth=3  IndexOptions=Index vector (dialog)  Indices=[1]  OutputSizes=1
  Selector1 : Selector  InputPortWidth=3  IndexOptions=Index vector (dialog)  Indices=[1]  OutputSizes=1
  Series RLC Branch2 : powerlib/Elements/Series RLC Branch  LConnTagsString=__new0  RConnTagsString=__new0  BranchType=L  Resistance=1  Inductance=15e-6  SetiL0=off  InitialCurrent=0  Capacitance=1e-6  Setx0=off  InitialVoltage=0  Measurements=None
      settings: SourceProductName=Simscape Electrical
  Series RLC Branch3 : powerlib/Elements/Series RLC Branch  Commented=on  LConnTagsString=__new0  RConnTagsString=__new0  BranchType=R  Resistance=10  Inductance=1e-3  SetiL0=off  InitialCurrent=0  Capacitance=C  Setx0=off  InitialVoltage=400  Measurements=None
      settings: SourceProductName=Simscape Electrical
  Series RLC Branch4 : powerlib/Elements/Series RLC Branch  LConnTagsString=__new0  RConnTagsString=__new0  BranchType=RC  Resistance=0.1  Inductance=1e-3  SetiL0=off  InitialCurrent=0  Capacitance=C  Setx0=off  InitialVoltage=400  Measurements=None
      settings: SourceProductName=Simscape Electrical
  Subsystem : Subsystem
  Subsystem1 : Subsystem
  Subsystem2 : Subsystem
  Subsystem3 : Subsystem
  Subsystem4 : Subsystem
  Subsystem7 : Subsystem
  Subsystem8 : Subsystem
  Sum1 : Sum  Inputs=|-+
  Sum2 : Sum  Inputs=|-+
  Sum4 : Sum  Inputs=|-+
  Terminator : Terminator
  Terminator1 : Terminator
  Terminator2 : Terminator
  VSC (Average Model) : powerlib/Power Electronics/Universal Bridge  Arms=3  SnubberResistance=1e5  SnubberCapacitance=inf  Device=Average-model based VSC  Ron=1e-3  Lon=0  ForwardVoltages="[  0  0  ]"  ForwardVoltage=0  GTOparameters=[ 10e-6 , 20e-6 ]  IGBTparameters=[ 1e-6 , 2e-6 ]  Measurements=None  Measurements_2=None  converterType=Rectifier
      settings: SourceProductName=Simscape Electrical
  VSC (Average Model)3 : powerlib/Power Electronics/Universal Bridge  Arms=2  SnubberResistance=1e5  SnubberCapacitance=inf  Device=Average-model based VSC  Ron=1e-3  Lon=0  ForwardVoltages="[  0  0  ]"  ForwardVoltage=0  GTOparameters=[ 10e-6 , 20e-6 ]  IGBTparameters=[ 1e-6 , 2e-6 ]  Measurements=None  Measurements_2=None  converterType=Rectifier
      settings: SourceProductName=Simscape Electrical
  VSC (Average Model)4 : powerlib/Power Electronics/Universal Bridge  Arms=2  SnubberResistance=1e5  SnubberCapacitance=inf  Device=Average-model based VSC  Ron=1e-3  Lon=0  ForwardVoltages="[  0  0  ]"  ForwardVoltage=0  GTOparameters=[ 10e-6 , 20e-6 ]  IGBTparameters=[ 1e-6 , 2e-6 ]  Measurements=None  Measurements_2=None  converterType=Rectifier
      settings: SourceProductName=Simscape Electrical
  V_I grid : Scope  NumInputPorts=2
  Vdc_bus2 : Scope
  Voltage Measurement2 : powerlib/Measurements/Voltage Measurement  PhasorSimulation=off  OutputType=Complex  PSBequivalent=0
      settings: SourceProductName=Simscape Electrical
  a : PMIOPort  Side=Right
  b : PMIOPort  Port=2  Side=Right
  c : PMIOPort  Port=3  Side=Right
  Qcap : Outport
  wires:
  Sum2/1 -> Subsystem4/1(e(S))  "e(S)"
  PLL (3ph)/2 -> Subsystem2/1(wt), Subsystem1/1(wt), Scope8/1, Subsystem/2(wt1)
  Mux1/1 -> Delay One Step/1
  Selector/1 -> V_I grid/1  "Va (V)"
  Delay One Step/1 -> Scope9/1, Subsystem/1(dq0)
  MATLAB Function1/1(id) -> Sum1/2
  Sum1/1 -> Subsystem3/1(e(S))  "e(S)"
  Subsystem4/1(u(S)) -> Mux1/2
  Power (Positive-Sequence)1/2 -> P_B2/2  "Q (kVA)"
  Demux/1 -> [Vd_C7]
  Pref/1 -> MATLAB Function1/1(P)
  [Iabc_B1_C7] -> Scope6/1, Subsystem2/2(abc)
  Subsystem/1(abc) -> Gain/1
  [Vabc_B2_C7] -> Selector/1, Power (Positive-Sequence)1/1
  Subsystem3/1(u(S)) -> Mux1/1
  Gain/1 -> Scope10/1, [Uref]
  Qref/1 -> MATLAB Function1/2(Q)
  [Vabc_B2_C7] -> Subsystem1/2(abc), PLL (3ph)/1
  Selector1/1 -> V_I grid/2  "Ia"
  Demux1/1 -> Sum1/1
  [Uref] -> VSC (Average Model)/1
  Demux/2 -> Terminator1/1
  [Iabc_B1_C7] -> Power (Positive-Sequence)1/2, Selector1/1
  Constant1/1 -> Mux1/3
  Subsystem1/1(dq) -> Demux/1, Scope4/1
  Demux1/2 -> Sum2/1
  Power (Positive-Sequence)1/1 -> P_B2/1  "P (kW)"
  MATLAB Function1/2(iq) -> Sum2/2
  [Vd_C7] -> MATLAB Function1/3(vd)
  PLL (3ph)/1 -> Terminator/1
  Subsystem2/1(dq) -> Demux1/1, Scope5/1
  B1/1 -> [Vabc_B2_C7]
  B1/2 -> [Iabc_B1_C7]
  Clock/1 -> MATLAB Function/1(u)
  Mean/1 -> Scope1/2, Sum4/1
  Constant6/1 -> Sum4/2
  [Vdc_DAB] -> Scope1/1, Mean/1
  Subsystem7/1(Uref_DAB1) -> Scope2/1, VSC (Average Model)4/1
  Subsystem7/2(Uref_DAB2) -> Scope2/2, VSC (Average Model)3/1
  Voltage Measurement2/1 -> Vdc_bus2/1, [Vdc_DAB]
  Sum4/1 -> Subsystem8/1(e)
  Subsystem8/1(u) -> Subsystem7/1(phase shift (-90,90))
  Battery1/1 -> Terminator2/1  "Battery"
  Constant/1 -> Qcap/1
  connections:
  VSC (Average Model)/LConn3 -- L/LConn3
  L/RConn1 -- B1/LConn1
  VSC (Average Model)/LConn1 -- L/LConn1
  L/RConn2 -- B1/LConn2
  VSC (Average Model)/LConn2 -- L/LConn2
  L/RConn3 -- B1/LConn3
  c/RConn1 -- B1/RConn3
  B1/RConn1 -- a/RConn1
  B1/RConn2 -- b/RConn1
  Series RLC Branch4/LConn1 -- DC Voltage Source2/RConn1 -- VSC (Average Model)4/RConn1 -- Series RLC Branch3/LConn1 -- VSC (Average Model)/RConn1 -- Voltage Measurement2/LConn1
  Series RLC Branch4/RConn1 -- VSC (Average Model)4/RConn2 -- DC Voltage Source2/LConn1 -- Series RLC Branch3/RConn1 -- Voltage Measurement2/LConn2 -- VSC (Average Model)/RConn2
  Linear Transformer1/RConn1 -- VSC (Average Model)4/LConn1
  Battery1/LConn1 -- VSC (Average Model)3/RConn1
  Series RLC Branch2/LConn1 -- VSC (Average Model)3/LConn1
  VSC (Average Model)3/RConn2 -- Battery1/LConn2
  Linear Transformer1/RConn2 -- VSC (Average Model)4/LConn2
  Series RLC Branch2/RConn1 -- Linear Transformer1/LConn1
  Linear Transformer1/LConn2 -- VSC (Average Model)3/LConn2
